simulink model "controlador_izaje"  (R2019a)
settings: Solver=VariableStepAuto  StartTime=0.0  StopTime=120  RelTol=1e-3
InitFcn:
  | parametros
undefined symbols (not defined in the file): b_cx, b_cy, b_h_eq, b_hb, b_hEb, b_t, b_t_eq, b_tb, b_td_eq, b_tw, b_wu, g, H_c, i_h, i_t, K_cy, K_d_h, K_d_t, K_i_h, K_i_t, k_p3_th, K_p_h, K_p_t, k_th, K_tw, k_w_c_th, k_wu, l_h0, L_h0, M_c_max, M_c_min, m_h_eq, M_s, M_t, m_td_eq, overload, r_hd, r_td, sigbuilder_block, T_hb_max, T_hEb_max, T_hm_MAX, T_s2, T_tb_max, T_tm_max, tau_hm, tau_tm, v_h_max, W_c, w_hm_rated, x_l0, x_t0, x_t_max_emer, x_t_max_oper, x_t_min_emer, x_t_min_oper, x_td0, xi_c_th, y_h_max_emer, y_h_max_oper ... (+4)
libraries: simulink x10
(part 1 of 2)
settings Model: Creator=Facundo  LastModifiedBy=Facundo

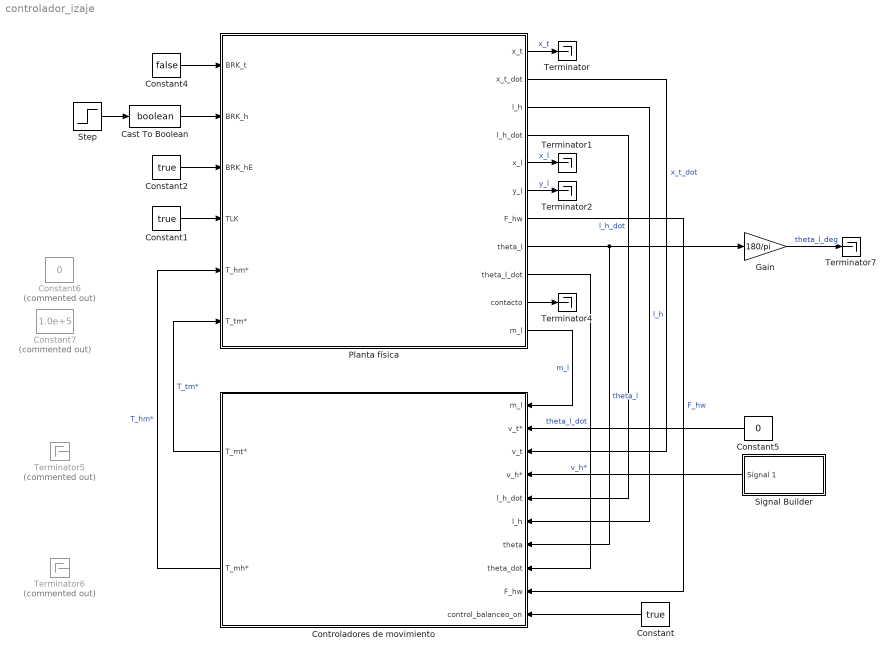
== system controlador_izaje ==
  Cast To Boolean : DataTypeConversion  OutDataTypeStr=boolean
  Constant : Constant  Value=true  OutDataTypeStr=boolean
  Constant1 : Constant  Value=true  OutDataTypeStr=boolean
  Constant2 : Constant  Value=true  OutDataTypeStr=boolean
  Constant4 : Constant  Value=false  OutDataTypeStr=boolean
  Constant5 : Constant  Value=0  OutDataTypeStr=boolean
  Constant6 : Constant  Commented=on  Value=0  OutDataTypeStr=double
  Constant7 : Constant  Commented=on  Value=1.0e+5  OutDataTypeStr=double
  Controladores de movimiento : Subsystem
  Gain : Gain  Gain=180/pi
  Planta física : Subsystem
  Signal Builder : Subsystem  Tag=STV Subsys  LoadFcn=sigbuilder_block('load');  StartFcn=sigbuilder_block('start');  StopFcn=sigbuilder_block('stop');  ClipboardFcn=sigbuilder_block('clipboard');  mask(Sigbuilder block){tuvar=[0:10]}
      mask help: Simulink:masks:SigbuilderBlock_MD
      mask init:
      | if ~strcmp(get_param(bdroot(gcbh),'SimulationStatus'),'stopped') tuvar = sigbuilder_block('maskInit'); end
      settings: CopyFcn=sigbuilder_block('copy');  DeleteFcn=sigbuilder_block('delete');  ModelCloseFcn=sigbuilder_block('modelClose');  PreSaveFcn=sigbuilder_block('preSave');  PauseFcn=sigbuilder_block('pause');  ContinueFcn=sigbuilder_block('continue');  NameChangeFcn=sigbuilder_block('namechange');  OpenFcn=sigbuilder_block('open',[5.14286 5.14286 812.571 450.429 ]);  CloseFcn=sigbuilder_block('close');
      mask Display: plot(0, 0, 100, 100,[2, 2, 32, 32, 2], [68, 8, 8, 68, 68],[32, 2], [38, 38], [32, 19, 2],[53, 60, 44], [32, 17, 17, 2],[16, 16, 31, 31]);txt = getActiveGroup(gcbh);text(2, 100, txt,'verticalAlignment', 'top');
  Step : Step  Time=80  Before=1  After=0  SampleTime=0
  Terminator{,1..2,4,7} (5 alike) : Terminator
  Terminator5 : Terminator  Commented=on
  Terminator6 : Terminator  Commented=on
  wires:
  Constant/1 -> Controladores de movimiento/10(control_balanceo_on)
  Controladores de movimiento/1(T_mt*) -> Planta física/6(T_tm*)  "T_tm*"
  Controladores de movimiento/2(T_mh*) -> Planta física/5(T_hm*)  "T_hm*"
  Planta física/2(x_t_dot) -> Controladores de movimiento/3(v_t)  "x_t_dot"
  Planta física/4(l_h_dot) -> Controladores de movimiento/5(l_h_dot)  "l_h_dot"
  Planta física/8(theta_l) -> Gain/1, Controladores de movimiento/7(theta)  "theta_l"
  Planta física/9(theta_l_dot) -> Controladores de movimiento/8(theta_dot)  "theta_l_dot"
  Planta física/3(l_h) -> Controladores de movimiento/6(l_h)  "l_h"
  Planta física/1(x_t) -> Terminator/1  "x_t"
  Constant1/1 -> Planta física/4(TLK)
  Constant2/1 -> Planta física/3(BRK_hE)
  Cast To Boolean/1 -> Planta física/2(BRK_h)
  Constant4/1 -> Planta física/1(BRK_t)
  Planta física/5(x_l) -> Terminator1/1  "x_l"
  Planta física/6(y_l) -> Terminator2/1  "y_l"
  Planta física/7(F_hw) -> Controladores de movimiento/9(F_hw)  "F_hw"
  Planta física/10(contacto) -> Terminator4/1
  Planta física/11(m_l) -> Controladores de movimiento/1(m_l)  "m_l"
  Gain/1 -> Terminator7/1  "theta_l_deg"
  Signal Builder/1(Signal 1) -> Controladores de movimiento/4(v_h*)  "v_h*"
  Constant5/1 -> Controladores de movimiento/2(v_t*)
  Step/1 -> Cast To Boolean/1

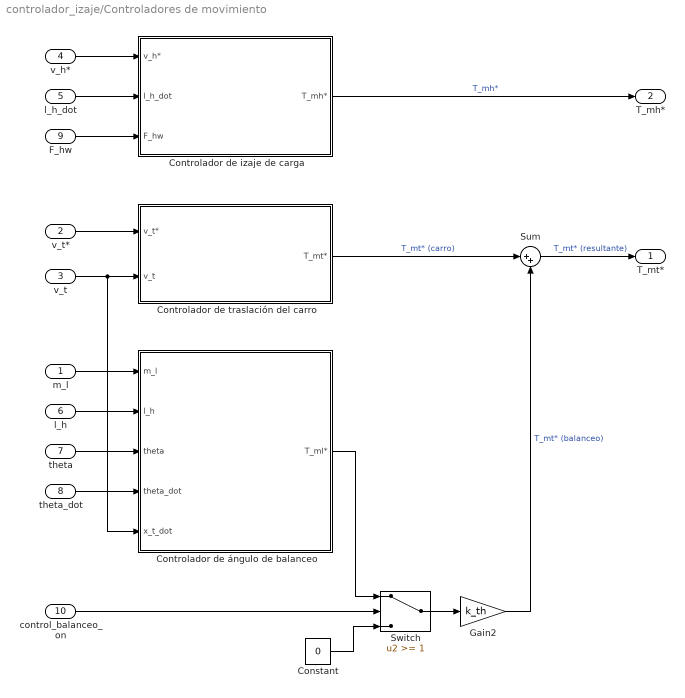
== system controlador_izaje/Controladores de movimiento ==
  m_l : Inport
  v_t* : Inport  Port=2
  v_t : Inport  Port=3
  v_h* : Inport  Port=4
  l_h_dot : Inport  Port=5
  l_h : Inport  Port=6
  theta : Inport  Port=7
  theta_dot : Inport  Port=8
  F_hw : Inport  Port=9
  control_balanceo_on : Inport  Port=10  OutDataTypeStr=boolean  LockScale=on
  Constant : Constant  Value=0
  Controlador de izaje de carga : Subsystem
  Controlador de traslación del carro : Subsystem
  Controlador de ángulo de balanceo : Subsystem
  Gain2 : Gain  Gain=k_th
  Sum : Sum  Inputs=|++
  Switch : Switch  Threshold=1
  T_mt* : Outport
  T_mh* : Outport  Port=2
  wires:
  v_t*/1 -> Controlador de traslación del carro/1(v_t*)
  Controlador de izaje de carga/1(T_mh*) -> T_mh*/1  "T_mh*"
  l_h_dot/1 -> Controlador de izaje de carga/2(l_h_dot)
  v_h*/1 -> Controlador de izaje de carga/1(v_h*)
  v_t/1 -> Controlador de ángulo de balanceo/5(x_t_dot), Controlador de traslación del carro/2(v_t)
  Controlador de traslación del carro/1(T_mt*) -> Sum/1  "T_mt* (carro)"
  Sum/1 -> T_mt*/1  "T_mt* (resultante)"
  Constant/1 -> Switch/3
  Switch/1 -> Gain2/1
  Controlador de ángulo de balanceo/1(T_ml*) -> Switch/1
  theta/1 -> Controlador de ángulo de balanceo/3(theta)
  l_h/1 -> Controlador de ángulo de balanceo/2(l_h)
  theta_dot/1 -> Controlador de ángulo de balanceo/4(theta_dot)
  control_balanceo_on/1 -> Switch/2
  m_l/1 -> Controlador de ángulo de balanceo/1(m_l)
  Gain2/1 -> Sum/2  "T_mt* (balanceo)"
  F_hw/1 -> Controlador de izaje de carga/3(F_hw)

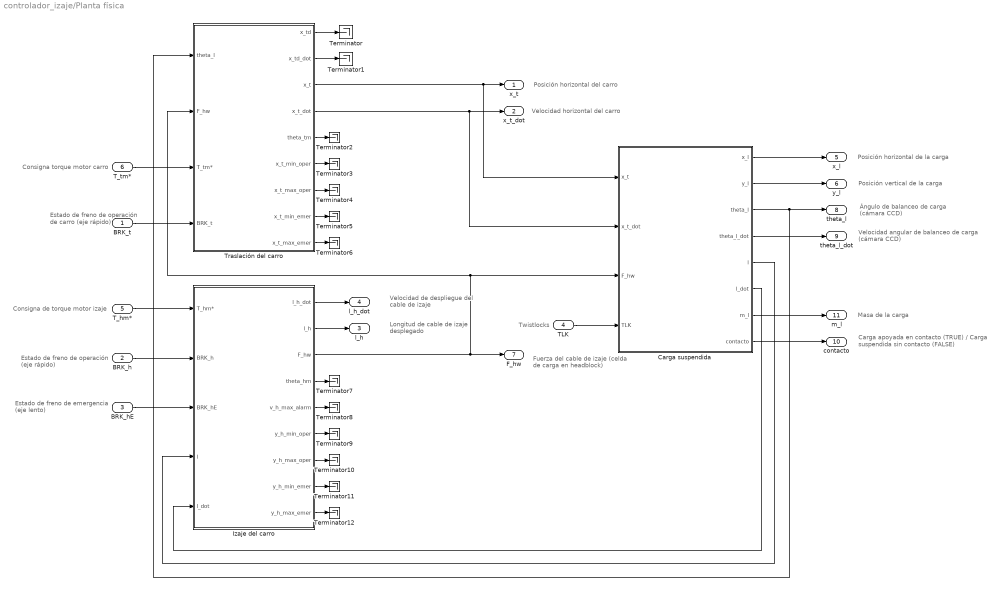
== system controlador_izaje/Planta física ==
  note: Consigna de torque motor izaje
  note: Posición horizontal del carro
  note: Velocidad de despliegue
      | del cable de izaje
  note: Longitud de cable
      | de izaje desplegado
  note: Posición horizontal de la carga
  note: Fuerza del cable de izaje
      | (celda de carga en headblock)
  note: Estado de freno de emergencia
      | (eje lento)
  note: Twistlocks
  note: Estado de freno de operación
      | (eje rápido)
  note: Ángulo de balanceo de carga
      | (cámara CCD)
  note: Consigna torque motor carro
  note: Estado de freno de
      | operación de carro
      | (eje rápido)
  note: Posición vertical de la carga
  note: Velocidad horizontal del carro
  note: Velocidad angular de balanceo de carga
      | (cámara CCD)
  note: Masa de la carga
  note: Carga apoyada en contacto (TRUE) /
      | Carga suspendida sin contacto (FALSE)
  BRK_t : Inport
  BRK_h : Inport  Port=2
  BRK_hE : Inport  Port=3
  TLK : Inport  Port=4  OutDataTypeStr=boolean  PortDimensions=1  SampleTime=0
  T_hm* : Inport  Port=5
  T_tm* : Inport  Port=6
  Carga suspendida : Subsystem
  Izaje del carro : Subsystem
  Terminator{,1..12} (13 alike) : Terminator
  Traslación del carro : Subsystem
  x_t : Outport
  x_t_dot : Outport  Port=2
  l_h : Outport  Port=3
  l_h_dot : Outport  Port=4
  x_l : Outport  Port=5
  y_l : Outport  Port=6
  F_hw : Outport  Port=7
  theta_l : Outport  Port=8
  theta_l_dot : Outport  Port=9
  contacto : Outport  Port=10
  m_l : Outport  Port=11
  wires:
  BRK_hE/1 -> Izaje del carro/3(BRK_hE)
  BRK_h/1 -> Izaje del carro/2(BRK_h)
  Traslación del carro/3(x_t) -> Carga suspendida/1(x_t), x_t/1
  BRK_t/1 -> Traslación del carro/4(BRK_t)
  Traslación del carro/1(x_td) -> Terminator/1
  Izaje del carro/1(l_h_dot) -> l_h_dot/1
  Izaje del carro/3(F_hw) -> F_hw/1, Traslación del carro/2(F_hw), Carga suspendida/3(F_hw)
  Carga suspendida/6(l_dot) -> Izaje del carro/5(l_dot)
  Carga suspendida/5(l) -> Izaje del carro/4(l)
  TLK/1 -> Carga suspendida/4(TLK)
  Carga suspendida/3(theta_l) -> Traslación del carro/1(theta_l), theta_l/1
  T_hm*/1 -> Izaje del carro/1(T_hm*)
  Carga suspendida/1(x_l) -> x_l/1
  Izaje del carro/2(l_h) -> l_h/1
  Carga suspendida/2(y_l) -> y_l/1
  Traslación del carro/4(x_t_dot) -> Carga suspendida/2(x_t_dot), x_t_dot/1
  Traslación del carro/2(x_td_dot) -> Terminator1/1
  T_tm*/1 -> Traslación del carro/3(T_tm*)
  Traslación del carro/5(theta_tm) -> Terminator2/1
  Traslación del carro/6(x_t_min_oper) -> Terminator3/1
  Traslación del carro/7(x_t_max_oper) -> Terminator4/1
  Traslación del carro/8(x_t_min_emer) -> Terminator5/1
  Traslación del carro/9(x_t_max_emer) -> Terminator6/1
  Izaje del carro/4(theta_hm) -> Terminator7/1
  Izaje del carro/5(v_h_max_alarm) -> Terminator8/1
  Izaje del carro/6(y_h_min_oper) -> Terminator9/1
  Izaje del carro/7(y_h_max_oper) -> Terminator10/1
  Izaje del carro/8(y_h_min_emer) -> Terminator11/1
  Izaje del carro/9(y_h_max_emer) -> Terminator12/1
  Carga suspendida/4(theta_l_dot) -> theta_l_dot/1
  Carga suspendida/8(contacto) -> contacto/1
  Carga suspendida/7(m_l) -> m_l/1

== system controlador_izaje/Signal Builder ==
  Demux : Demux  Tag=STV Demux  Outputs=1
  FromWs : FromWorkspace  Tag=STV FromWs  VariableName=tuvar  SampleTime=0
      SigBuilderData=|
      | common.afterFinalStr = 'Extrapolate'
      | common.sampleTime = 0
      | dataSet.timeRange = [0 60]
      | dataSet.name = 'Group 1'
      | sbobj.Groups.Name = 'Group 1'
      | sbobj.Groups.Signals.Name = 'Signal 1'
      | sbobj.Groups.Signals.XData = [0 5 15 35 45 60]
      | sbobj.Groups.Signals.YData = [0 0 1 1 0 0]
      | sbobj.Groups.TimeRange = [0 60]
  Signal 1 : Outport  Tag=STV Outport
  wires:
  FromWs/1 -> Demux/1
  Demux/1 -> Signal 1/1

== system controlador_izaje/Controladores de movimiento/Controlador de izaje de carga ==
  v_h* : Inport
  l_h_dot : Inport  Port=2
  F_hw : Inport  Port=3
  Gain : Gain  Gain=K_d_h
  Gain1 : Gain  Gain=-1
  Gain2 : Gain  Gain=K_p_h
  Gain3 : Gain  Gain=K_i_h
  Gain5 : Gain  Gain=r_hd/i_h
  Integrator : Integrator
  Integrator1 : Integrator
  Sum : Sum  Inputs=+++
  Sum1 : Sum  Inputs=|+-
  Sum2 : Sum  Inputs=|-+
  T_mh* : Outport
  wires:
  Integrator1/1 -> Gain3/1
  Gain/1 -> Sum/3  "acción D"
  v_h*/1 -> Gain1/1  "v_h*"
  Integrator/1 -> Gain2/1, Integrator1/1
  Gain3/1 -> Sum/1  "acción I"
  Gain2/1 -> Sum/2  "acción P"
  Sum/1 -> Sum2/1  "F_h_eq_total*"
  Sum1/1 -> Gain/1, Integrator/1  "e_l_h"
  Gain1/1 -> Sum1/1  "l_h_dot*"
  l_h_dot/1 -> Sum1/2  "l_h_dot"
  Gain5/1 -> T_mh*/1  "T_mh*"
  F_hw/1 -> Sum2/2  "F_hw"
  Sum2/1 -> Gain5/1

== system controlador_izaje/Controladores de movimiento/Controlador de traslación del carro ==
  v_t* : Inport
  v_t : Inport  Port=2
  Gain : Gain  Gain=K_d_t
  Gain1 : Gain  Gain=r_td/i_t
  Gain2 : Gain  Gain=K_p_t
  Gain3 : Gain  Gain=K_i_t
  Integrator : Integrator
  Integrator1 : Integrator
  Sum : Sum  Inputs=+++
  Sum1 : Sum  Inputs=|+-
  T_mt* : Outport
  wires:
  v_t/1 -> Sum1/2
  Integrator/1 -> Gain2/1, Integrator1/1
  Gain2/1 -> Sum/2  "acción P"
  Gain3/1 -> Sum/1  "acción I"
  Sum1/1 -> Gain/1, Integrator/1  "e_v_t"
  v_t*/1 -> Sum1/1
  Integrator1/1 -> Gain3/1
  Gain/1 -> Sum/3  "acción D"
  Sum/1 -> Gain1/1  "F_t_eq*"
  Gain1/1 -> T_mt*/1  "T_mt*"

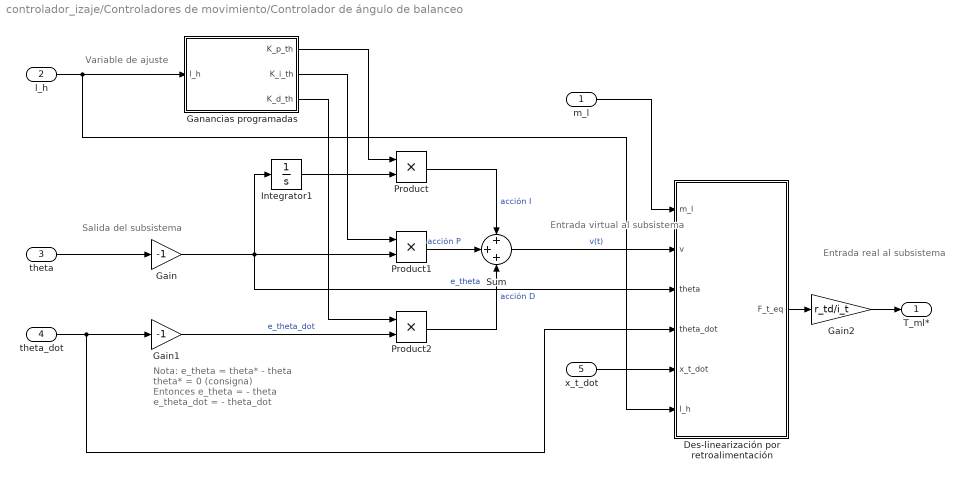
== system controlador_izaje/Controladores de movimiento/Controlador de ángulo de balanceo ==
  note: Entrada virtual
      | al subsistema
  note: Nota:
      | e_theta = theta* - theta
      | theta* = 0 (consigna)
      |
      | Entonces
      | e_theta = - theta
      | e_theta_dot = - theta_dot
  note: Variable de ajuste
  note: Salida del
      | subsistema
  note: Entrada real
      | al subsistema
  m_l : Inport
  l_h : Inport  Port=2
  theta : Inport  Port=3
  theta_dot : Inport  Port=4
  x_t_dot : Inport  Port=5
  Des-linearización por retroalimentación : Subsystem
  Gain : Gain  Gain=-1
  Gain1 : Gain  Gain=-1
  Gain2 : Gain  Gain=r_td/i_t
  Ganancias programadas : Subsystem
  Integrator1 : Integrator
  Product : Product
  Product1 : Product
  Product2 : Product
  Sum : Sum  Inputs=+++
  T_ml* : Outport
  wires:
  Product1/1 -> Sum/2  "acción P"
  Product/1 -> Sum/1  "acción I"
  Integrator1/1 -> Product/2
  Product2/1 -> Sum/3  "acción D"
  Ganancias programadas/1(K_p_th) -> Product/1
  Ganancias programadas/2(K_i_th) -> Product1/1
  Ganancias programadas/3(K_d_th) -> Product2/1
  l_h/1 -> Des-linearización por retroalimentación/6(l_h), Ganancias programadas/1(l_h)
  Gain1/1 -> Product2/2  "e_theta_dot"
  theta/1 -> Gain/1
  theta_dot/1 -> Des-linearización por retroalimentación/4(theta_dot), Gain1/1
  Sum/1 -> Des-linearización por retroalimentación/2(v)  "v(t)"
  x_t_dot/1 -> Des-linearización por retroalimentación/5(x_t_dot)
  Des-linearización por retroalimentación/1(F_t_eq) -> Gain2/1
  Gain2/1 -> T_ml*/1
  m_l/1 -> Des-linearización por retroalimentación/1(m_l)
  Gain/1 -> Product1/2, Des-linearización por retroalimentación/3(theta), Integrator1/1  "e_theta"

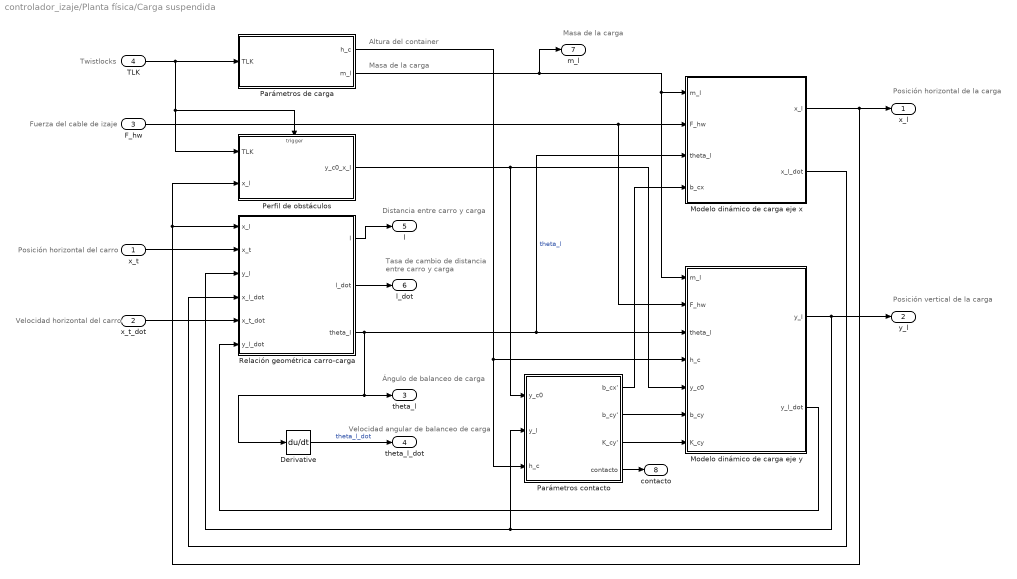
== system controlador_izaje/Planta física/Carga suspendida ==
  note: Masa de la carga
  note: Twistlocks
  note: Altura del container
  note: Posición horizontal del carro
  note: Posición vertical de la carga
  note: Velocidad horizontal del carro
  note: Distancia entre carro y carga
  note: Fuerza del cable de izaje
  note: Ángulo de balanceo de carga
  note: Tasa de cambio de distancia
      | entre carro y carga
  note: Masa de la carga
  note: Posición horizontal de la carga
  note: Velocidad angular de balanceo de carga
  x_t : Inport  OutDataTypeStr=double  PortDimensions=1  SampleTime=0
  x_t_dot : Inport  Port=2  OutDataTypeStr=double  PortDimensions=1  SampleTime=0
  F_hw : Inport  Port=3  OutDataTypeStr=double  PortDimensions=1  SampleTime=0
  TLK : Inport  Port=4  OutDataTypeStr=boolean  PortDimensions=1  SampleTime=0
  Derivative : Derivative
  Modelo dinámico de carga eje x : Subsystem
  Modelo dinámico de carga eje y : Subsystem
  Parámetros contacto : Subsystem
  Parámetros de carga : Subsystem
  Perfil de obstáculos : Subsystem
  Relación geométrica carro-carga : Subsystem
  x_l : Outport  OutDataTypeStr=double  PortDimensions=1  SampleTime=0
  y_l : Outport  Port=2  OutDataTypeStr=double  PortDimensions=1  SampleTime=0
  theta_l : Outport  Port=3  OutDataTypeStr=double  PortDimensions=1  SampleTime=0
  theta_l_dot : Outport  Port=4  OutDataTypeStr=double  PortDimensions=1  SampleTime=0
  l : Outport  Port=5  OutDataTypeStr=double  PortDimensions=1  SampleTime=0
  l_dot : Outport  Port=6  OutDataTypeStr=double  PortDimensions=1  SampleTime=0
  m_l : Outport  Port=7  OutDataTypeStr=double  PortDimensions=1  SampleTime=0
  contacto : Outport  Port=8  OutDataTypeStr=boolean  PortDimensions=1  SampleTime=0
  wires:
  Parámetros de carga/2(m_l) -> m_l/1, Modelo dinámico de carga eje y/1(m_l), Modelo dinámico de carga eje x/1(m_l)
  F_hw/1 -> Modelo dinámico de carga eje y/2(F_hw), Modelo dinámico de carga eje x/2(F_hw)
  Relación geométrica carro-carga/2(l_dot) -> l_dot/1
  x_t_dot/1 -> Relación geométrica carro-carga/5(x_t_dot)
  Modelo dinámico de carga eje y/1(y_l) -> y_l/1, Parámetros contacto/2(y_l), Relación geométrica carro-carga/3(y_l)
  Modelo dinámico de carga eje x/2(x_l_dot) -> Relación geométrica carro-carga/4(x_l_dot)
  Modelo dinámico de carga eje y/2(y_l_dot) -> Relación geométrica carro-carga/6(y_l_dot)
  x_t/1 -> Relación geométrica carro-carga/2(x_t)
  Modelo dinámico de carga eje x/1(x_l) -> Perfil de obstáculos/2(x_l), Relación geométrica carro-carga/1(x_l), x_l/1
  Relación geométrica carro-carga/3(theta_l) -> Derivative/1, theta_l/1, Modelo dinámico de carga eje x/3(theta_l), Modelo dinámico de carga eje y/3(theta_l)  "theta_l"
  Parámetros contacto/1(b_cx') -> Modelo dinámico de carga eje x/4(b_cx)
  Parámetros contacto/2(b_cy') -> Modelo dinámico de carga eje y/6(b_cy)
  Parámetros contacto/3(K_cy') -> Modelo dinámico de carga eje y/7(K_cy)
  Relación geométrica carro-carga/1(l) -> l/1
  Parámetros contacto/4(contacto) -> contacto/1
  Parámetros de carga/1(h_c) -> Modelo dinámico de carga eje y/4(h_c), Parámetros contacto/3(h_c)
  Perfil de obstáculos/1(y_c0_x_l) -> Parámetros contacto/1(y_c0), Modelo dinámico de carga eje y/5(y_c0)
  TLK/1 -> Parámetros de carga/1(TLK), Perfil de obstáculos/Trigger, Perfil de obstáculos/1(TLK)
  Derivative/1 -> theta_l_dot/1  "theta_l_dot"

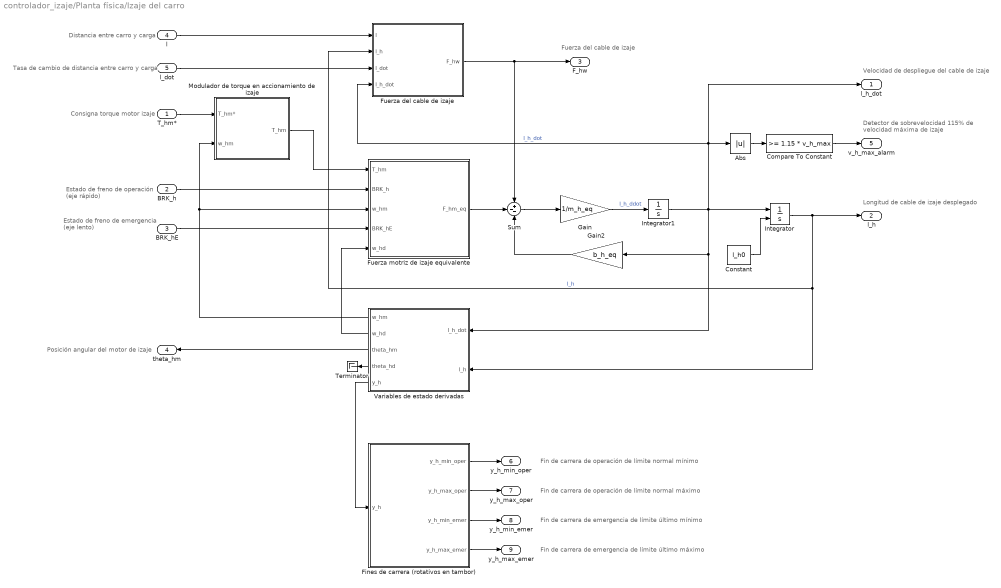
== system controlador_izaje/Planta física/Izaje del carro ==
  note: Detector de sobrevelocidad
      | 115% de velocidad máxima de izaje
  note: Posición angular del motor de izaje
  note: Longitud de cable de izaje desplegado
  note: Velocidad de despliegue del cable de izaje
  note: Consigna torque motor izaje
  note: Estado de freno de emergencia
      | (eje lento)
  note: Tasa de cambio de distancia entre carro y carga
  note: Estado de freno de operación
      | (eje rápido)
  note: Distancia entre carro y carga
  note: Fuerza del cable de izaje
  note: Fin de carrera de operación de límite normal mínimo
  note: Fin de carrera de emergencia de límite último máximo
  note: Fin de carrera de emergencia de límite último mínimo
  note: Fin de carrera de operación de límite normal máximo
  T_hm* : Inport
  BRK_h : Inport  Port=2
  BRK_hE : Inport  Port=3
  l : Inport  Port=4
  l_dot : Inport  Port=5
  Abs : Abs
  Compare To Constant : simulink/Logic and Bit Operations/Compare To Constant  relop=>=  const=1.15 * v_h_max  OutDataTypeStr=boolean
  Constant : Constant  Value=l_h0
  Fines de carrera (rotativos en tambor) : Subsystem
  Fuerza del cable de izaje : Subsystem
  Fuerza motriz de izaje equivalente : Subsystem
  Gain : Gain  Gain=1/m_h_eq
  Gain2 : Gain  Gain=b_h_eq
  Integrator : Integrator  InitialConditionSource=external
  Integrator1 : Integrator
  Modulador de torque en accionamiento de izaje : Subsystem
  Sum : Sum  Inputs=+--
  Terminator : Terminator
  Variables de estado derivadas : Subsystem
  l_h_dot : Outport
  l_h : Outport  Port=2
  F_hw : Outport  Port=3
  theta_hm : Outport  Port=4
  v_h_max_alarm : Outport  Port=5
  y_h_min_oper : Outport  Port=6  OutDataTypeStr=boolean  PortDimensions=1  SampleTime=0
  y_h_max_oper : Outport  Port=7  OutDataTypeStr=boolean  PortDimensions=1  SampleTime=0
  y_h_min_emer : Outport  Port=8  OutDataTypeStr=boolean  PortDimensions=1  SampleTime=0
  y_h_max_emer : Outport  Port=9  OutDataTypeStr=boolean  PortDimensions=1  SampleTime=0
  wires:
  Integrator/1 -> l_h/1, Variables de estado derivadas/2(l_h), Fuerza del cable de izaje/2(l_h)  "l_h"
  Integrator1/1 -> l_h_dot/1, Fuerza del cable de izaje/4(l_h_dot), Abs/1, Variables de estado derivadas/1(l_h_dot), Gain2/1, Integrator/1  "l_h_dot"
  l/1 -> Fuerza del cable de izaje/1(l)
  l_dot/1 -> Fuerza del cable de izaje/3(l_dot)
  Fuerza del cable de izaje/1(F_hw) -> F_hw/1, Sum/1
  Gain2/1 -> Sum/3
  Fuerza motriz de izaje equivalente/1(F_hm_eq) -> Sum/2
  Variables de estado derivadas/1(w_hm) -> Fuerza motriz de izaje equivalente/3(w_hm), Modulador de torque en accionamiento de izaje/2(w_hm)
  Sum/1 -> Gain/1
  Variables de estado derivadas/2(w_hd) -> Fuerza motriz de izaje equivalente/5(w_hd)
  BRK_h/1 -> Fuerza motriz de izaje equivalente/2(BRK_h)
  BRK_hE/1 -> Fuerza motriz de izaje equivalente/4(BRK_hE)
  Gain/1 -> Integrator1/1  "l_h_ddot"
  Constant/1 -> Integrator/2
  Variables de estado derivadas/3(theta_hm) -> theta_hm/1
  Abs/1 -> Compare To Constant/1
  Compare To Constant/1 -> v_h_max_alarm/1
  Fines de carrera (rotativos en tambor)/1(y_h_min_oper) -> y_h_min_oper/1
  Fines de carrera (rotativos en tambor)/4(y_h_max_emer) -> y_h_max_emer/1
  Fines de carrera (rotativos en tambor)/3(y_h_min_emer) -> y_h_min_emer/1
  Fines de carrera (rotativos en tambor)/2(y_h_max_oper) -> y_h_max_oper/1
  Variables de estado derivadas/5(y_h) -> Fines de carrera (rotativos en tambor)/1(y_h)
  Variables de estado derivadas/4(theta_hd) -> Terminator/1
  Modulador de torque en accionamiento de izaje/1(T_hm) -> Fuerza motriz de izaje equivalente/1(T_hm)
  T_hm*/1 -> Modulador de torque en accionamiento de izaje/1(T_hm*)

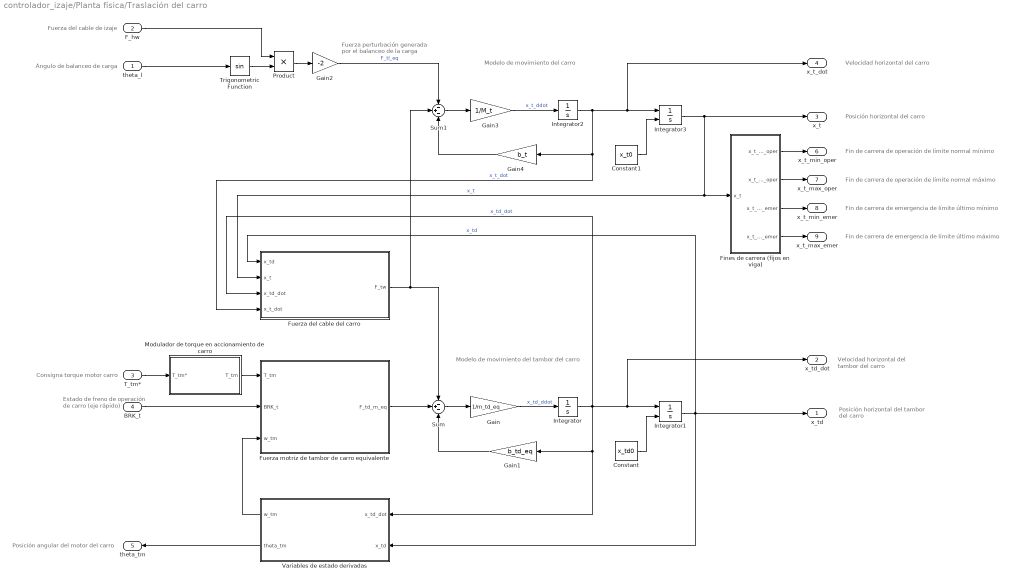
== system controlador_izaje/Planta física/Traslación del carro ==
  note: Posición angular del motor del carro
  note: Velocidad horizontal
      | del tambor del carro
  note: Modelo de movimiento del tambor del carro
  note: Modelo de movimiento del carro
  note: Velocidad horizontal del carro
  note: Estado de freno de
      | operación de carro
      | (eje rápido)
  note: Fuerza del cable de izaje
  note: Fuerza perturbación generada
      | por el balanceo de la carga
  note: Posición horizontal del carro
  note: Consigna torque motor carro
  note: Ángulo de balanceo de carga
  note: Posición horizontal
      | del tambor del carro
  note: Fin de carrera de operación de límite normal mínimo
  note: Fin de carrera de operación de límite normal máximo
  note: Fin de carrera de emergencia de límite último mínimo
  note: Fin de carrera de emergencia de límite último máximo
  theta_l : Inport  OutDataTypeStr=double  PortDimensions=1  SampleTime=0
  F_hw : Inport  Port=2  OutDataTypeStr=double  PortDimensions=1  SampleTime=0
  T_tm* : Inport  Port=3
  BRK_t : Inport  Port=4
  Constant : Constant  Value=x_td0
  Constant1 : Constant  Value=x_t0
  Fines de carrera (fijos en viga) : Subsystem
  Fuerza del cable del carro : Subsystem
  Fuerza motriz de tambor de carro equivalente : Subsystem
  Gain : Gain  Gain=1/m_td_eq
  Gain1 : Gain  Gain=b_td_eq
  Gain2 : Gain  Gain=-2
  Gain3 : Gain  Gain=1/M_t
  Gain4 : Gain  Gain=b_t
  Integrator : Integrator
  Integrator1 : Integrator  InitialConditionSource=external
  Integrator2 : Integrator
  Integrator3 : Integrator  InitialConditionSource=external
  Modulador de torque en accionamiento de carro : Subsystem
  Product : Product
  Sum : Sum  Inputs=-+-
  Sum1 : Sum  Inputs=-+-
  Trigonometric Function : Trigonometry
  Variables de estado derivadas : Subsystem
  x_td : Outport  OutDataTypeStr=double  PortDimensions=1  SampleTime=0
  x_td_dot : Outport  Port=2  OutDataTypeStr=double  PortDimensions=1  SampleTime=0
  x_t : Outport  Port=3  OutDataTypeStr=double  PortDimensions=1  SampleTime=0
  x_t_dot : Outport  Port=4  OutDataTypeStr=double  PortDimensions=1  SampleTime=0
  theta_tm : Outport  Port=5  OutDataTypeStr=double  PortDimensions=1  SampleTime=0
  x_t_min_oper : Outport  Port=6  OutDataTypeStr=boolean  PortDimensions=1  SampleTime=0
  x_t_max_oper : Outport  Port=7  OutDataTypeStr=boolean  PortDimensions=1  SampleTime=0
  x_t_min_emer : Outport  Port=8  OutDataTypeStr=boolean  PortDimensions=1  SampleTime=0
  x_t_max_emer : Outport  Port=9  OutDataTypeStr=boolean  PortDimensions=1  SampleTime=0
  wires:
  Integrator1/1 -> Variables de estado derivadas/2(x_td), Fuerza del cable del carro/1(x_td), x_td/1  "x_td"
  Gain3/1 -> Integrator2/1  "x_t_ddot"
  Fuerza del cable del carro/1(F_tw) -> Sum1/2, Sum/1
  Sum/1 -> Gain/1
  Integrator/1 -> Fuerza del cable del carro/3(x_td_dot), Variables de estado derivadas/1(x_td_dot), Gain1/1, x_td_dot/1, Integrator1/1  "x_td_dot"
  F_hw/1 -> Product/1
  Fuerza motriz de tambor de carro equivalente/1(F_td_m_eq) -> Sum/2
  Constant/1 -> Integrator1/2
  Gain1/1 -> Sum/3
  Integrator2/1 -> Fuerza del cable del carro/4(x_t_dot), Gain4/1, x_t_dot/1, Integrator3/1  "x_t_dot"
  Sum1/1 -> Gain3/1
  theta_l/1 -> Trigonometric Function/1
  Gain4/1 -> Sum1/3
  Integrator3/1 -> x_t/1, Fuerza del cable del carro/2(x_t), Fines de carrera (fijos en viga)/1(x_t)  "x_t"
  Gain2/1 -> Sum1/1  "F_tl_eq"
  T_tm*/1 -> Modulador de torque en accionamiento de carro/1(T_tm*)
  BRK_t/1 -> Fuerza motriz de tambor de carro equivalente/2(BRK_t)
  Variables de estado derivadas/1(w_tm) -> Fuerza motriz de tambor de carro equivalente/3(w_tm)
  Constant1/1 -> Integrator3/2
  Trigonometric Function/1 -> Product/2
  Product/1 -> Gain2/1
  Gain/1 -> Integrator/1  "x_td_ddot"
  Variables de estado derivadas/2(theta_tm) -> theta_tm/1
  Fines de carrera (fijos en viga)/1(x_t_min_oper) -> x_t_min_oper/1
  Fines de carrera (fijos en viga)/2(x_t_max_oper) -> x_t_max_oper/1
  Fines de carrera (fijos en viga)/3(x_t_min_emer) -> x_t_min_emer/1
  Fines de carrera (fijos en viga)/4(x_t_max_emer) -> x_t_max_emer/1
  Modulador de torque en accionamiento de carro/1(T_tm) -> Fuerza motriz de tambor de carro equivalente/1(T_tm)

== system controlador_izaje/Controladores de movimiento/Controlador de ángulo de balanceo/Des-linearización por retroalimentación ==
  note: Linearización por retroalimentación (feedback linearization)
      | F_t_eq = ( v - a ) / b
      | Siendo v la entrada virtual al sistema lineal a controlar
  m_l : Inport
  v : Inport  Port=2
  theta : Inport  Port=3
  theta_dot : Inport  Port=4
  x_t_dot : Inport  Port=5
  l_h : Inport  Port=6
  Add : Sum  Inputs=+-
  Divide : Product  Inputs=*/
  MATLAB Function : MATLAB Function  TreatAsAtomicUnit=on
  MATLAB Function1 : MATLAB Function  TreatAsAtomicUnit=on
  F_t_eq : Outport
  wires:
  Add/1 -> Divide/1
  v/1 -> Add/1
  Divide/1 -> F_t_eq/1
  MATLAB Function/1(a) -> Add/2
  MATLAB Function1/1(b) -> Divide/2
  theta/1 -> MATLAB Function1/1(theta), MATLAB Function/1(theta)
  theta_dot/1 -> MATLAB Function/2(theta_dot)
  x_t_dot/1 -> MATLAB Function/3(x_t_dot)
  l_h/1 -> MATLAB Function1/2(l_h), MATLAB Function/4(l_h)
  m_l/1 -> MATLAB Function/5(m_l), MATLAB Function1/3(m_l)

== system controlador_izaje/Controladores de movimiento/Controlador de ángulo de balanceo/Ganancias programadas ==
  note: Ganancia proporcional K_p_th
      | K_p_th = w_c_th^2 + 2*xi_c_th*w_c_th*p3_th
  note: Ganancia derivativa K_d_th
      | K_d_th = 2*xi_c_th*w_c_th + p3_th
  note: Ganancia integral K_i_th
      | K_i_th = p3_th*w_c_th^2
  l_h : Inport
  Add : Sum
  Add1 : Sum
  Gain : Gain  Gain=2*xi_c_th
  Gain1 : Gain  Gain=2*xi_c_th
  Parametros deseados sistema a lazo cerrado : Subsystem
  Product : Product
  Product1 : Product
  Product2 : Product  Inputs=3
  K_p_th : Outport
  K_i_th : Outport  Port=2
  K_d_th : Outport  Port=3
  wires:
  l_h/1 -> Parametros deseados sistema a lazo cerrado/1(l_h)
  Parametros deseados sistema a lazo cerrado/1(w_c_th) -> Product2/3, Product2/2, Product/2, Product/1, Product1/1, Gain1/1
  Parametros deseados sistema a lazo cerrado/2(p3_th) -> Product2/1, Product1/2, Add1/2
  Product1/1 -> Gain/1
  Gain/1 -> Add/2
  Product/1 -> Add/1
  Add/1 -> K_p_th/1  "K_p_th"
  Gain1/1 -> Add1/1
  Add1/1 -> K_d_th/1  "K_d_th"
  Product2/1 -> K_i_th/1  "K_i_th"

== system controlador_izaje/Planta física/Carga suspendida/Modelo dinámico de carga eje x ==
  note: Componente horizontal de
      | fuerza del cable de izaje
  note: Posición horizontal de la carga
  note: Velocidad horizontal de la carga
  note: Fuerza del cable de izaje
  note: Masa de la carga
  note: Fricción por contacto
      | horizontal (arrastre)
  note: Ángulo de balanceo de carga
  m_l : Inport  OutDataTypeStr=double  PortDimensions=1  SampleTime=0
  F_hw : Inport  Port=2  OutDataTypeStr=double  PortDimensions=1  SampleTime=0
  theta_l : Inport  Port=3  OutDataTypeStr=double  PortDimensions=1  SampleTime=0
  b_cx : Inport  Port=4  OutDataTypeStr=double  PortDimensions=1  SampleTime=0
  Constant : Constant  Value=x_l0
  Divide : Product  Inputs=*/
  Gain2 : Gain  Gain=-2
  Integrator : Integrator
  Integrator1 : Integrator  InitialConditionSource=external
  Product : Product
  Product1 : Product
  Sum : Sum  Inputs=|+-
  Trigonometric Function : Trigonometry
  x_l : Outport  OutDataTypeStr=double  PortDimensions=1  SampleTime=0
  x_l_dot : Outport  Port=2  OutDataTypeStr=double  PortDimensions=1  SampleTime=0
  wires:
  F_hw/1 -> Product/1
  Product1/1 -> Sum/2
  theta_l/1 -> Trigonometric Function/1
  b_cx/1 -> Product1/2
  Sum/1 -> Divide/1
  Integrator/1 -> x_l_dot/1, Integrator1/1, Product1/1  "x_l_dot"
  Product/1 -> Gain2/1
  Divide/1 -> Integrator/1  "x_l_ddot"
  Constant/1 -> Integrator1/2
  Integrator1/1 -> x_l/1
  Gain2/1 -> Sum/1
  m_l/1 -> Divide/2
  Trigonometric Function/1 -> Product/2

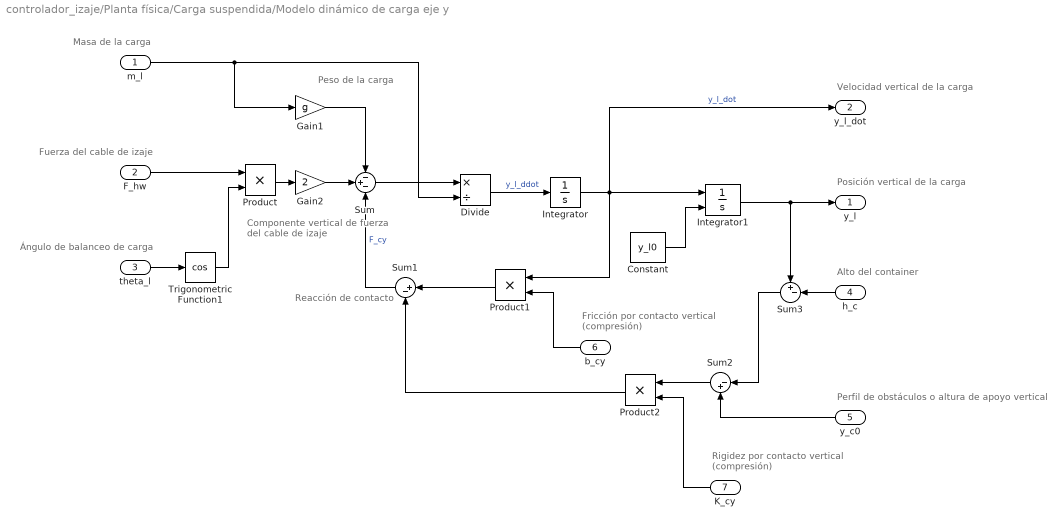
== system controlador_izaje/Planta física/Carga suspendida/Modelo dinámico de carga eje y ==
  note: Reacción de contacto
  note: Peso de la carga
  note: Componente vertical de
      | fuerza del cable de izaje
  note: Posición vertical de la carga
  note: Velocidad vertical de la carga
  note: Fricción por contacto
      | vertical (compresión)
  note: Rigidez por contacto
      | vertical (compresión)
  note: Masa de la carga
  note: Fuerza del cable de izaje
  note: Perfil de obstáculos o altura de apoyo vertical
  note: Alto del container
  note: Ángulo de balanceo de carga
  m_l : Inport  OutDataTypeStr=double  PortDimensions=1  SampleTime=0
  F_hw : Inport  Port=2  OutDataTypeStr=double  PortDimensions=1  SampleTime=0
  theta_l : Inport  Port=3  OutDataTypeStr=double  PortDimensions=1  SampleTime=0
  h_c : Inport  Port=4  OutDataTypeStr=double  PortDimensions=1  SampleTime=0
  y_c0 : Inport  Port=5  OutDataTypeStr=double  PortDimensions=1  SampleTime=0
  b_cy : Inport  Port=6  OutDataTypeStr=double  PortDimensions=1  SampleTime=0
  K_cy : Inport  Port=7  OutDataTypeStr=double  PortDimensions=1  SampleTime=0
  Constant : Constant  Value=y_l0
  Divide : Product  Inputs=*/
  Gain1 : Gain  Gain=g
  Gain2 : Gain  Gain=2
  Integrator : Integrator
  Integrator1 : Integrator  InitialConditionSource=external
  Product : Product
  Product1 : Product
  Product2 : Product
  Sum : Sum  Inputs=-+-
  Sum1 : Sum  Inputs=|+-
  Sum2 : Sum  Inputs=|-+
  Sum3 : Sum  Inputs=+-|
  Trigonometric Function1 : Trigonometry  Operator=cos
  y_l : Outport  OutDataTypeStr=double  PortDimensions=1  SampleTime=0
  y_l_dot : Outport  Port=2  OutDataTypeStr=double  PortDimensions=1  SampleTime=0
  wires:
  F_hw/1 -> Product/1
  theta_l/1 -> Trigonometric Function1/1
  b_cy/1 -> Product1/2
  Integrator/1 -> y_l_dot/1, Integrator1/1, Product1/1  "y_l_dot"
  Divide/1 -> Integrator/1  "y_l_ddot"
  Constant/1 -> Integrator1/2
  Integrator1/1 -> y_l/1, Sum3/1
  Product/1 -> Gain2/1
  Product1/1 -> Sum1/1
  Sum1/1 -> Sum/3  "F_cy"
  Gain1/1 -> Sum/1
  y_c0/1 -> Sum2/2
  Sum2/1 -> Product2/1
  K_cy/1 -> Product2/2
  Product2/1 -> Sum1/2
  Gain2/1 -> Sum/2
  Sum/1 -> Divide/1
  m_l/1 -> Gain1/1, Divide/2
  h_c/1 -> Sum3/2
  Sum3/1 -> Sum2/1
  Trigonometric Function1/1 -> Product/2

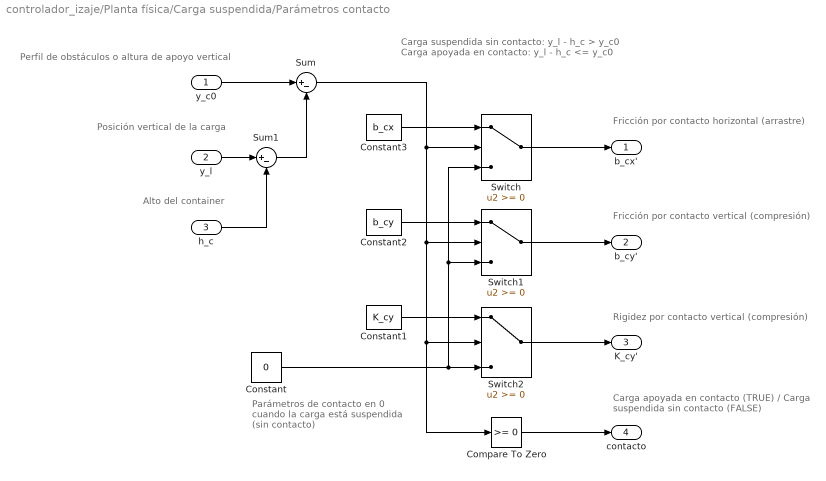
== system controlador_izaje/Planta física/Carga suspendida/Parámetros contacto ==
  note: Fricción por contacto horizontal (arrastre)
  note: Fricción por contacto vertical (compresión)
  note: Rigidez por contacto vertical (compresión)
  note: Perfil de obstáculos o altura de apoyo vertical
  note: Posición vertical de la carga
  note: Alto del container
  note: Parámetros de contacto en 0
      | cuando la carga está suspendida
      | (sin contacto)
  note: Carga suspendida sin contacto: y_l - h_c > y_c0
      | Carga apoyada en contacto: y_l - h_c <= y_c0
  note: Carga apoyada en contacto (TRUE) /
      | Carga suspendida sin contacto (FALSE)
  y_c0 : Inport  OutDataTypeStr=double  PortDimensions=1  SampleTime=0
  y_l : Inport  Port=2  OutDataTypeStr=double  PortDimensions=1  SampleTime=0
  h_c : Inport  Port=3  OutDataTypeStr=double  PortDimensions=1  SampleTime=0
  Compare To Zero : simulink/Logic and Bit Operations/Compare To Zero  relop=>=  OutDataTypeStr=boolean
  Constant : Constant  Value=0
  Constant1 : Constant  Value=K_cy
  Constant2 : Constant  Value=b_cy
  Constant3 : Constant  Value=b_cx
  Sum : Sum  Inputs=|+-
  Sum1 : Sum  Inputs=|+-
  Switch : Switch
  Switch1 : Switch
  Switch2 : Switch
  b_cx' : Outport  OutDataTypeStr=double  PortDimensions=1  SampleTime=0
  b_cy' : Outport  Port=2  OutDataTypeStr=double  PortDimensions=1  SampleTime=0
  K_cy' : Outport  Port=3  OutDataTypeStr=double  PortDimensions=1  SampleTime=0
  contacto : Outport  Port=4  OutDataTypeStr=boolean  PortDimensions=1  SampleTime=0
  wires:
  y_c0/1 -> Sum/1
  Constant2/1 -> Switch1/1
  Constant1/1 -> Switch2/1
  Switch/1 -> b_cx'/1
  Sum/1 -> Switch1/2, Compare To Zero/1, Switch2/2, Switch/2
  Switch2/1 -> K_cy'/1
  Switch1/1 -> b_cy'/1
  Constant/1 -> Switch/3, Switch1/3, Switch2/3
  Constant3/1 -> Switch/1
  Sum1/1 -> Sum/2
  y_l/1 -> Sum1/1
  h_c/1 -> Sum1/2
  Compare To Zero/1 -> contacto/1

== system controlador_izaje/Planta física/Carga suspendida/Parámetros de carga ==
  note: Twistlocks
  note: Masa de la carga total
  note: Alto del container
      | (afecta altura inferior)
  note: Masa del spreader
  note: Masa del contenedor
      | y carga
  TLK : Inport  OutDataTypeStr=boolean  PortDimensions=1  SampleTime=0
  "Generate random load " : Subsystem  TreatAsAtomicUnit=on
  Sum : Sum  Inputs=++|
  Switch : Switch  Criteria=u2 ~= 0
  Switch1 : Switch  Criteria=u2 ~= 0
  h_c1 : Constant  Value=H_c
  h_c2 : Constant  Value=0
  h_c3 : Constant  Value=M_s
  h_c4 : Constant  Value=0
  h_c : Outport
  m_l : Outport  Port=2
  wires:
  TLK/1 -> "Generate random load "/Trigger, Switch1/2, Switch/2
  Switch/1 -> h_c/1
  Sum/1 -> m_l/1
  Switch1/1 -> Sum/2  "M_cx"
  "Generate random load "/1(M_cx) -> Switch1/1
  h_c3/1 -> Sum/1  "M_s"
  h_c2/1 -> Switch/3
  h_c4/1 -> Switch1/3
  h_c1/1 -> Switch/1

== system controlador_izaje/Planta física/Carga suspendida/Perfil de obstáculos ==
  note: Perfil de obstáculos para x_l
  note: Se actualiza el perfil de obstá culos cuando
      | se cierran (TLK ↑) o abren (TLK ↓) los twistlocks
  note: Perfil de obstáculos
  note: Guarda perfil de obstáculos en workspace
      | para posterior análisis (plot_perfil_obstaculos.m)
  TLK : Inport  PortDimensions=1
  x_l : Inport  Port=2  OutDataTypeStr=double  PortDimensions=1
  Trigger : TriggerPort  TriggerType=either  VariantControl=Variant  PortDimensions=1
  MATLAB Function : MATLAB Function  TreatAsAtomicUnit=on
  To Workspace : ToWorkspace  VariableName=y_c0  SaveFormat=Structure With Time  SampleTime=-1
  y_c0_x_l : Outport  OutDataTypeStr=double  PortDimensions=1  InitialOutput=y_h_min_oper
  wires:
  MATLAB Function/1(y_c0_x_l) -> y_c0_x_l/1
  TLK/1 -> MATLAB Function/2(TLK)
  x_l/1 -> MATLAB Function/1(x_l)
  MATLAB Function/2(y_c0) -> To Workspace/1

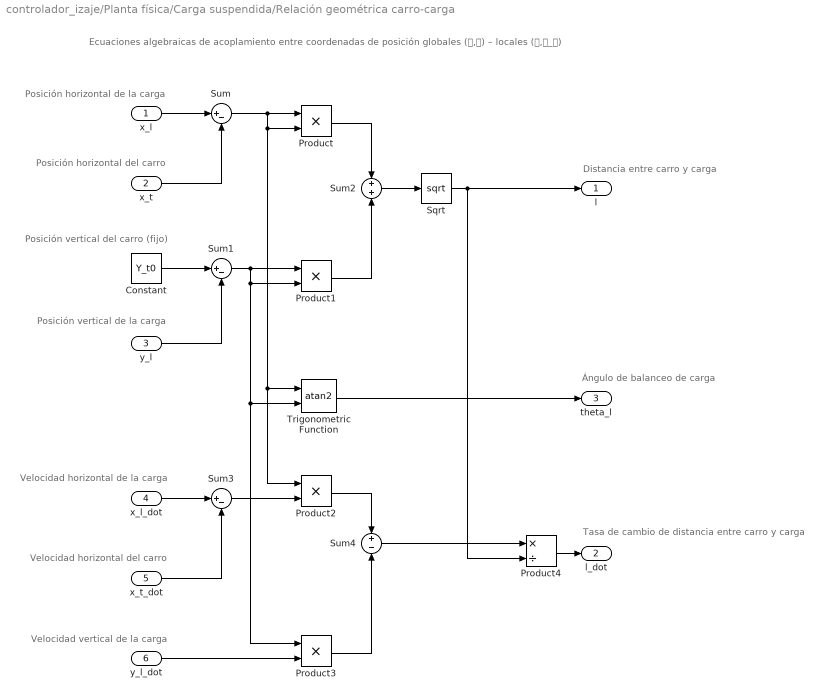
== system controlador_izaje/Planta física/Carga suspendida/Relación geométrica carro-carga ==
  note: Ecuaciones algebraicas de acoplamiento entre coordenadas de posición globales (𝑥,𝑦) – locales (𝑙,𝜃_𝑙)
  note: Posición horizontal de la carga
  note: Posición horizontal del carro
  note: Posición vertical del carro (fijo)
  note: Posición vertical de la carga
  note: Distancia entre carro y carga
  note: Tasa de cambio de distancia entre carro y carga
  note: Ángulo de balanceo de carga
  note: Velocidad horizontal de la carga
  note: Velocidad horizontal del carro
  note: Velocidad vertical de la carga
  x_l : Inport
  x_t : Inport  Port=2
  y_l : Inport  Port=3
  x_l_dot : Inport  Port=4
  x_t_dot : Inport  Port=5
  y_l_dot : Inport  Port=6
  Constant : Constant  Value=Y_t0
  Product{,1..3} (4 alike) : Product
  Product4 : Product  Inputs=*/
  Sqrt : Sqrt  SaturateOnIntegerOverflow=on
  Sum : Sum  Inputs=|+-
  Sum1 : Sum  Inputs=|+-
  Sum2 : Sum  Inputs=+|+
  Sum3 : Sum  Inputs=|+-
  Sum4 : Sum  Inputs=+|-
  Trigonometric Function : Trigonometry  Operator=atan2
  l : Outport
  l_dot : Outport  Port=2
  theta_l : Outport  Port=3
  wires:
  x_t/1 -> Sum/2
  x_l/1 -> Sum/1
  Sum/1 -> Product/1, Product2/1, Trigonometric Function/1, Product/2
  Product/1 -> Sum2/1
  y_l/1 -> Sum1/2
  Sum1/1 -> Product1/1, Product3/1, Trigonometric Function/2, Product1/2
  Constant/1 -> Sum1/1
  Product1/1 -> Sum2/2
  Sum2/1 -> Sqrt/1
  Trigonometric Function/1 -> theta_l/1
  x_l_dot/1 -> Sum3/1
  x_t_dot/1 -> Sum3/2
  Sum3/1 -> Product2/2
  y_l_dot/1 -> Product3/2
  Product2/1 -> Sum4/1
  Product3/1 -> Sum4/2
  Sum4/1 -> Product4/1
  Product4/1 -> l_dot/1
  Sqrt/1 -> Product4/2, l/1

== system controlador_izaje/Planta física/Izaje del carro/Fines de carrera (rotativos en tambor) ==
  note: Fines de carrera son rotativos sobre tambor (theta_hd). Por simplicidad se usa la variable equivalente lineal (y_h)
  note: Fin de carrera de operación de límite normal mínimo
  note: Fin de carrera de operación de límite normal máximo
  note: Fin de carrera de emergencia de límite último mínimo
  note: Fin de carrera de operación de límite último máximo
  note: Altura de la carga sin balanceo
  y_h : Inport
  Compare To Constant : simulink/Logic and Bit Operations/Compare To Constant  relop=<=  const=y_h_min_oper  OutDataTypeStr=boolean
  Compare To Constant1 : simulink/Logic and Bit Operations/Compare To Constant  relop=>=  const=y_h_max_oper  OutDataTypeStr=boolean
  Compare To Constant2 : simulink/Logic and Bit Operations/Compare To Constant  relop=<=  const=y_h_min_emer  OutDataTypeStr=boolean
  Compare To Constant3 : simulink/Logic and Bit Operations/Compare To Constant  relop=>=  const=y_h_max_emer  OutDataTypeStr=boolean
  y_h_min_oper : Outport  OutDataTypeStr=boolean  PortDimensions=1  SampleTime=0
  y_h_max_oper : Outport  Port=2  OutDataTypeStr=boolean  PortDimensions=1  SampleTime=0
  y_h_min_emer : Outport  Port=3  OutDataTypeStr=boolean  PortDimensions=1  SampleTime=0
  y_h_max_emer : Outport  Port=4  OutDataTypeStr=boolean  PortDimensions=1  SampleTime=0
  wires:
  Compare To Constant2/1 -> y_h_min_emer/1
  Compare To Constant/1 -> y_h_min_oper/1
  Compare To Constant1/1 -> y_h_max_oper/1
  y_h/1 -> Compare To Constant3/1, Compare To Constant2/1, Compare To Constant1/1, Compare To Constant/1
  Compare To Constant3/1 -> y_h_max_emer/1

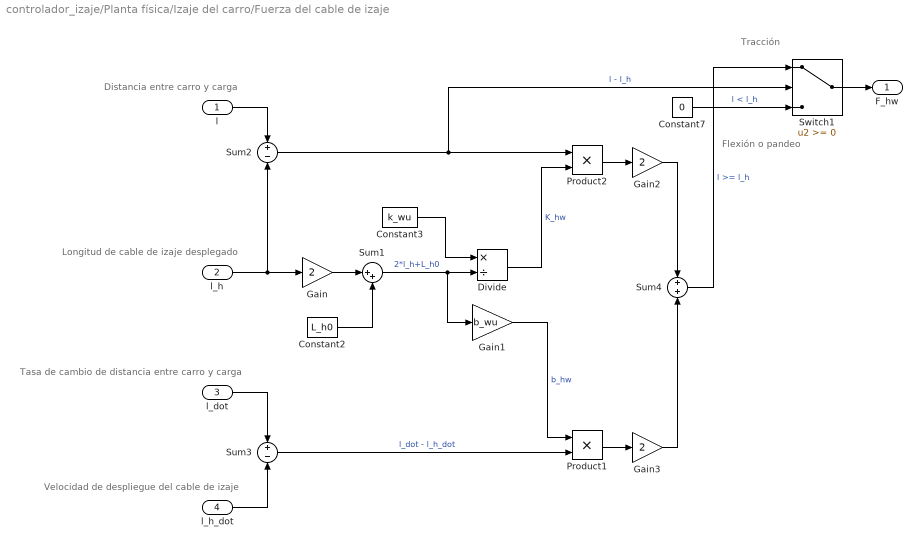
== system controlador_izaje/Planta física/Izaje del carro/Fuerza del cable de izaje ==
  note: Flexión o pandeo
  note: Tracción
  note: Distancia entre carro y carga
  note: Tasa de cambio de distancia entre carro y carga
  note: Longitud de cable de izaje desplegado
  note: Velocidad de despliegue del cable de izaje
  l : Inport
  l_h : Inport  Port=2
  l_dot : Inport  Port=3
  l_h_dot : Inport  Port=4
  Constant2 : Constant  Value=L_h0
  Constant3 : Constant  Value=k_wu
  Constant7 : Constant  Value=0
  Divide : Product  Inputs=*/
  Gain : Gain  Gain=2
  Gain1 : Gain  Gain=b_wu
  Gain2 : Gain  Gain=2
  Gain3 : Gain  Gain=2
  Product1 : Product
  Product2 : Product
  Sum1 : Sum  Inputs=|++
  Sum2 : Sum  Inputs=+-
  Sum3 : Sum  Inputs=+-
  Sum4 : Sum
  Switch1 : Switch
  F_hw : Outport
  wires:
  l_dot/1 -> Sum3/1
  Constant2/1 -> Sum1/2
  Sum1/1 -> Gain1/1, Divide/2  "2*l_h+L_h0"
  l/1 -> Sum2/1
  Product1/1 -> Gain3/1
  Sum3/1 -> Product1/2  "l_dot - l_h_dot"
  l_h_dot/1 -> Sum3/2
  l_h/1 -> Gain/1, Sum2/2
  Divide/1 -> Product2/2  "K_hw"
  Sum2/1 -> Switch1/2, Product2/1  "l - l_h"
  Constant3/1 -> Divide/1
  Gain1/1 -> Product1/1  "b_hw"
  Product2/1 -> Gain2/1
  Switch1/1 -> F_hw/1
  Sum4/1 -> Switch1/1  "l >= l_h"
  Constant7/1 -> Switch1/3  "l < l_h"
  Gain/1 -> Sum1/1
  Gain2/1 -> Sum4/1
  Gain3/1 -> Sum4/2

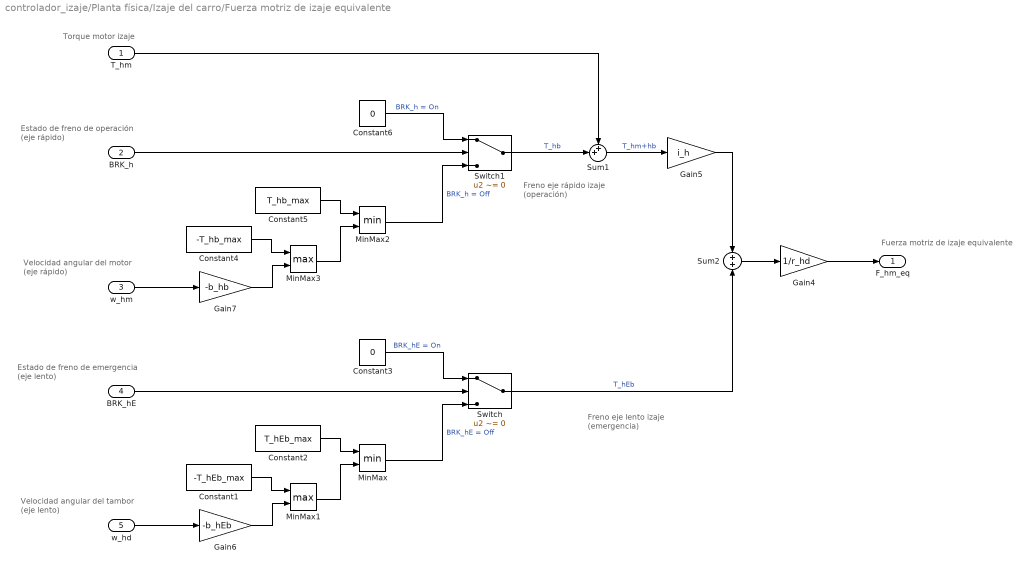
== system controlador_izaje/Planta física/Izaje del carro/Fuerza motriz de izaje equivalente ==
  note: Fuerza motriz de izaje equivalente
  note: Torque motor izaje
  note: Freno eje lento izaje
      | (emergencia)
  note: Freno eje rápido izaje
      | (operación)
  note: Estado de freno de operación
      | (eje rápido)
  note: Estado de freno de emergencia
      | (eje lento)
  note: Velocidad angular del tambor
      | (eje lento)
  note: Velocidad angular del motor
      | (eje rápido)
  T_hm : Inport
  BRK_h : Inport  Port=2  OutDataTypeStr=boolean
  w_hm : Inport  Port=3
  BRK_hE : Inport  Port=4  OutDataTypeStr=boolean
  w_hd : Inport  Port=5
  Constant1 : Constant  Value=-T_hEb_max
  Constant2 : Constant  Value=T_hEb_max
  Constant3 : Constant  Value=0
  Constant4 : Constant  Value=-T_hb_max
  Constant5 : Constant  Value=T_hb_max
  Constant6 : Constant  Value=0
  Gain4 : Gain  Gain=1/r_hd
  Gain5 : Gain  Gain=i_h
  Gain6 : Gain  Gain=-b_hEb
  Gain7 : Gain  Gain=-b_hb
  MinMax : MinMax  Inputs=2
  MinMax1 : MinMax  Function=max  Inputs=2
  MinMax2 : MinMax  Inputs=2
  MinMax3 : MinMax  Function=max  Inputs=2
  Sum1 : Sum  Inputs=++|
  Sum2 : Sum  Inputs=2
  Switch : Switch  Criteria=u2 ~= 0
  Switch1 : Switch  Criteria=u2 ~= 0
  F_hm_eq : Outport
  wires:
  MinMax3/1 -> MinMax2/2
  MinMax1/1 -> MinMax/2
  Constant1/1 -> MinMax1/1
  MinMax2/1 -> Switch1/3  "BRK_h = Off"
  Gain5/1 -> Sum2/1
  Constant4/1 -> MinMax3/1
  T_hm/1 -> Sum1/1
  w_hm/1 -> Gain7/1
  Constant5/1 -> MinMax2/1
  w_hd/1 -> Gain6/1
  Gain7/1 -> MinMax3/2
  BRK_h/1 -> Switch1/2
  Constant6/1 -> Switch1/1  "BRK_h = On"
  MinMax/1 -> Switch/3  "BRK_hE = Off"
  Sum1/1 -> Gain5/1  "T_hm+hb"
  Switch1/1 -> Sum1/2  "T_hb"
  Constant3/1 -> Switch/1  "BRK_hE = On"
  BRK_hE/1 -> Switch/2
  Constant2/1 -> MinMax/1
  Gain6/1 -> MinMax1/2
  Gain4/1 -> F_hm_eq/1
  Sum2/1 -> Gain4/1
  Switch/1 -> Sum2/2  "T_hEb"

== system controlador_izaje/Planta física/Izaje del carro/Modulador de torque en accionamiento de izaje ==
  note: Modelo de torque idealizado equivalente,
      | modelo simplificado de primer orden LTI en tiempo continuo
  note: Consigna de torque de motor de izaje
  note: Velocidad del motor de izaje
  note: Torque de motor de izaje
  T_hm* : Inport
  w_hm : Inport  Port=2
  Gain1 : Gain  Gain=1/tau_hm
  Gain3 : Gain  Gain=-1
  Integrator2 : Integrator
  Limitador de torque máximo en tiempo discretizado : Subsystem
  Reducción cuadrática de torque máximo (field weakening) : Subsystem
  Sum : Sum  Inputs=|++
  T_hm : Outport
  wires:
  Integrator2/1 -> T_hm/1, Gain3/1  "T_hm"
  Gain3/1 -> Sum/2
  Gain1/1 -> Integrator2/1  "T_hm_dot"
  Sum/1 -> Gain1/1
  Limitador de torque máximo en tiempo discretizado/1(T_hm_lim*) -> Sum/1  "T_hm_lim*"
  Reducción cuadrática de torque máximo (field weakening)/1(T_hm_max) -> Limitador de torque máximo en tiempo discretizado/1(T_hm_max)  "T_hm_max"
  T_hm*/1 -> Limitador de torque máximo en tiempo discretizado/2(T_hm*)  "T_hm*"
  w_hm/1 -> Reducción cuadrática de torque máximo (field weakening)/1(w_hm)  "w_hm"

== system controlador_izaje/Planta física/Izaje del carro/Variables de estado derivadas ==
  note: Velocidad angular del tambor
  note: Caja reductora
      | entre motor y tambor
  note: Velocidad angular del motor
  note: Velocidad de despliegue del cable de izaje
  note: Longitud de cable de izaje desplegado
  note: Posición angular del motor
  note: Caja reductora
      | entre motor y tambor
  note: Radio del tambor
  note: Radio del tambor
  note: Normalizar ángulo en
      | rango 0 a 2*pi
  note: Posición angular del tambor
  note: Altura de carro (fija)
  note: Altura de la carga sin balanceo
  l_h_dot : Inport
  l_h : Inport  Port=2
  Constant1 : Constant  Value=2*pi
  Constant2 : Constant  Value=Y_t0
  Gain1 : Gain  Gain=-2/r_hd
  Gain2 : Gain  Gain=-2/r_hd
  Gain3 : Gain  Gain=i_h
  Gain4 : Gain  Gain=i_h
  Mod2 : Math  Operator=mod  SaturateOnIntegerOverflow=on
  Sum : Sum  Inputs=+-|
  w_hm : Outport
  w_hd : Outport  Port=2
  theta_hm : Outport  Port=3
  theta_hd : Outport  Port=4
  y_h : Outport  Port=5
  wires:
  Gain1/1 -> w_hd/1, Gain3/1  "w_hd"
  l_h_dot/1 -> Gain1/1
  Gain3/1 -> w_hm/1  "w_hm"
  Gain2/1 -> theta_hd/1, Gain4/1  "theta_hd"
  l_h/1 -> Sum/2, Gain2/1
  Gain4/1 -> Mod2/1  "theta_hm_raw"
  Constant1/1 -> Mod2/2
  Mod2/1 -> theta_hm/1
  Constant2/1 -> Sum/1
  Sum/1 -> y_h/1  "y_h"

== system controlador_izaje/Planta física/Traslación del carro/Fines de carrera (fijos en viga) ==
  note: Posición horizontal del carro
  note: Fin de carrera de operación de límite normal mínimo
  note: Fin de carrera de operación de límite normal máximo
  note: Fin de carrera de emergencia de límite último mínimo
  note: Fin de carrera de operación de límite último máximo
  x_t : Inport
  Compare To Constant : simulink/Logic and Bit Operations/Compare To Constant  relop=<=  const=x_t_min_oper  OutDataTypeStr=boolean
  Compare To Constant1 : simulink/Logic and Bit Operations/Compare To Constant  relop=>=  const=x_t_max_oper  OutDataTypeStr=boolean
  Compare To Constant2 : simulink/Logic and Bit Operations/Compare To Constant  relop=<=  const=x_t_min_emer  OutDataTypeStr=boolean
  Compare To Constant3 : simulink/Logic and Bit Operations/Compare To Constant  relop=>=  const=x_t_max_emer  OutDataTypeStr=boolean
  x_t_min_oper : Outport  OutDataTypeStr=boolean  PortDimensions=1  SampleTime=0
  x_t_max_oper : Outport  Port=2  OutDataTypeStr=boolean  PortDimensions=1  SampleTime=0
  x_t_min_emer : Outport  Port=3  OutDataTypeStr=boolean  PortDimensions=1  SampleTime=0
  x_t_max_emer : Outport  Port=4  OutDataTypeStr=boolean  PortDimensions=1  SampleTime=0
  wires:
  Compare To Constant2/1 -> x_t_min_emer/1
  Compare To Constant/1 -> x_t_min_oper/1
  Compare To Constant1/1 -> x_t_max_oper/1
  x_t/1 -> Compare To Constant3/1, Compare To Constant2/1, Compare To Constant1/1, Compare To Constant/1
  Compare To Constant3/1 -> x_t_max_emer/1

== system controlador_izaje/Planta física/Traslación del carro/Fuerza del cable del carro ==
  note: Posición de tambor del carro
  note: Velocidad del tambor del carro
  note: Posición del carro
  note: Velocidad del carro
  note: Fuerza del cable del carro
  x_td : Inport
  x_t : Inport  Port=2
  x_td_dot : Inport  Port=3
  x_t_dot : Inport  Port=4
  Gain : Gain  Gain=K_tw
  Gain1 : Gain  Gain=b_tw
  Sum2 : Sum  Inputs=+-
  Sum3 : Sum  Inputs=+-
  Sum4 : Sum
  F_tw : Outport
  wires:
  x_td_dot/1 -> Sum3/1
  x_td/1 -> Sum2/1
  x_t_dot/1 -> Sum3/2
  x_t/1 -> Sum2/2
  Sum4/1 -> F_tw/1
  Gain/1 -> Sum4/1
  Sum2/1 -> Gain/1
  Gain1/1 -> Sum4/2
  Sum3/1 -> Gain1/1

== system controlador_izaje/Planta física/Traslación del carro/Fuerza motriz de tambor de carro equivalente ==
  note: Fuerza motriz de tambor
      | de carro equivalente
  note: Torque motor carro
  note: Freno eje rápido izaje
      | (operación)
  note: Estado de freno de
      | operación de carro
      | (eje rápido)
  note: Velocidad angular
      | del motor de carro
      | (eje rápido)
  T_tm : Inport
  BRK_t : Inport  Port=2  OutDataTypeStr=boolean
  w_tm : Inport  Port=3
  Constant4 : Constant  Value=-T_tb_max
  Constant5 : Constant  Value=T_tb_max
  Constant6 : Constant  Value=0
  Gain4 : Gain  Gain=i_t/r_td
  Gain7 : Gain  Gain=-b_tb
  MinMax2 : MinMax  Inputs=2
  MinMax3 : MinMax  Function=max  Inputs=2
  Sum1 : Sum  Inputs=++|
  Switch1 : Switch  Criteria=u2 ~= 0
  F_td_m_eq : Outport
  wires:
  MinMax3/1 -> MinMax2/2
  MinMax2/1 -> Switch1/3  "BRK_t = Off"
  Constant4/1 -> MinMax3/1
  T_tm/1 -> Sum1/1
  w_tm/1 -> Gain7/1
  Constant5/1 -> MinMax2/1
  Gain7/1 -> MinMax3/2
  BRK_t/1 -> Switch1/2
  Constant6/1 -> Switch1/1  "BRK_t = On"
  Sum1/1 -> Gain4/1
  Switch1/1 -> Sum1/2  "T_tb"
  Gain4/1 -> F_td_m_eq/1

== system controlador_izaje/Planta física/Traslación del carro/Modulador de torque en accionamiento de carro ==
  note: Modelo de torque idealizado equivalente,
      | modelo simplificado de primer orden LTI en tiempo continuo
  note: Consigna de torque de motor de carro
  note: Torque de motor de carro
  T_tm* : Inport
  Gain1 : Gain  Gain=1/tau_tm
  Gain3 : Gain  Gain=-1
  Integrator2 : Integrator
  Limitador de torque máximo en tiempo discretizado : Subsystem
  Sum : Sum  Inputs=|++
  T_tm : Outport
  wires:
  Sum/1 -> Gain1/1
  Gain3/1 -> Sum/2
  Gain1/1 -> Integrator2/1  "T_tm_dot"
  Limitador de torque máximo en tiempo discretizado/1(T_tm_lim*) -> Sum/1  "T_tm_lim*"
  T_tm*/1 -> Limitador de torque máximo en tiempo discretizado/1(T_tm*)
  Integrator2/1 -> T_tm/1, Gain3/1  "T_tm"

== system controlador_izaje/Planta física/Traslación del carro/Variables de estado derivadas ==
  note: Normalizar ángulo en
      | rango 0 a 2*pi
  note: Radio del tambor
  note: Caja reductora
      | entre motor y tambor
  note: Velocidad angular del motor del carro
  note: Velocidad de la carga sin balanceo
  note: Posición angular del motor del carro
  note: Caja reductora
      | entre motor y tambor
  note: Radio del tambor
  note: Posición horizontal
      | del tambor del carro
  x_td_dot : Inport
  x_td : Inport  Port=2
  Constant : Constant  Value=2*pi
  Gain1 : Gain  Gain=1/r_td
  Gain2 : Gain  Gain=1/r_td
  Gain3 : Gain  Gain=i_t
  Gain4 : Gain  Gain=i_t
  Mod1 : Math  Operator=mod  SaturateOnIntegerOverflow=on
  w_tm : Outport
  theta_tm : Outport  Port=2
  wires:
  Gain1/1 -> Gain3/1  "w_td"
  x_td_dot/1 -> Gain1/1
  Gain3/1 -> w_tm/1  "w_tm"
  x_td/1 -> Gain2/1
  Gain2/1 -> Gain4/1  "theta_td"
  Gain4/1 -> Mod1/1  "theta_tm_raw"
  Mod1/1 -> theta_tm/1
  Constant/1 -> Mod1/2

== system controlador_izaje/Controladores de movimiento/Controlador de ángulo de balanceo/Ganancias programadas/Parametros deseados sistema a lazo cerrado ==
  note: Largo del cable de izaje
  note: Tercer polo de sistema a lazo cerrado
  note: Frecuencia natural del sistema a lazo cerrado
  l_h : Inport
  Constant : Constant  Value=k_w_c_th*sqrt(g)
  Divide : Product  Inputs=*/
  Gain : Gain  Gain=k_p3_th
  Sqrt : Sqrt  SaturateOnIntegerOverflow=on
  w_c_th : Outport
  p3_th : Outport  Port=2
  wires:
  Constant/1 -> Divide/1
  l_h/1 -> Sqrt/1
  Divide/1 -> w_c_th/1, Gain/1
  Sqrt/1 -> Divide/2
  Gain/1 -> p3_th/1

== system controlador_izaje/Planta física/Carga suspendida/Parámetros de carga/Generate random load  ==
  note: Masa de contenedor
      | Condiciones nominales: M_c_min <= M_cx <= M_c_max
      | Condición de sobrecarga: M_cx > M_c_max
  note: Condición de sobrecarga
  note: Masa del contenedor y carga
  note: Se actualiza la masa del contenedor de carga
      | cuando se cierran los twistlocks (TL K ↑)
  Trigger : TriggerPort  VariantControl=Variant  PortDimensions=1
  Constant : Constant  Value=M_c_min
  Constant1 : Constant  Value=M_c_max
  Constant2 : Constant  Value=1.25 * M_c_max
  Constant4 : Constant  Value=M_c_max
  MATLAB Function : MATLAB Function  TreatAsAtomicUnit=on
  Switch1 : Switch  Criteria=u2 ~= 0
  Switch2 : Switch  Criteria=u2 ~= 0
  h_c5 : Constant  Value=overload
  M_cx : Outport  OutDataTypeStr=double  PortDimensions=1  InitialOutput=0
  wires:
  MATLAB Function/1(y) -> M_cx/1
  Constant/1 -> Switch1/3
  Constant1/1 -> Switch1/1
  Constant2/1 -> Switch2/1
  Constant4/1 -> Switch2/3
  h_c5/1 -> Switch1/2, Switch2/2
  Switch1/1 -> MATLAB Function/1(min)
  Switch2/1 -> MATLAB Function/2(max)

== system controlador_izaje/Planta física/Izaje del carro/Modulador de torque en accionamiento de izaje/Limitador de torque máximo en tiempo discretizado ==
  note: Torque de motor de izaje máximo
      | con reducción cuadrática
  note: Consigna de torque de motor de izaje
  note: Consigna de torque de motor de izaje
      | con limitación de torque máximo
  note: Modelo discretizado
      | k * T_s2 <= t < (k+1) * T_s2
  T_hm_max : Inport
  T_hm* : Inport  Port=2
  Gain : Gain  Gain=-1
  MinMax : MinMax  Inputs=2
  MinMax1 : MinMax  Function=max  Inputs=2
  Zero-Order Hold : ZeroOrderHold  SampleTime=T_s2
  Zero-Order Hold1 : ZeroOrderHold  SampleTime=T_s2
  T_hm_lim* : Outport
  wires:
  T_hm*/1 -> Zero-Order Hold/1
  MinMax/1 -> Zero-Order Hold1/1
  T_hm_max/1 -> MinMax/1, Gain/1
  Gain/1 -> MinMax1/1
  MinMax1/1 -> MinMax/2
  Zero-Order Hold/1 -> MinMax1/2
  Zero-Order Hold1/1 -> T_hm_lim*/1
